simulink model "joint_trajectories"  (R2022a)
settings: Solver=FixedStepAuto  StartTime=0.0  StopTime=inf  RelTol=1e-3
libraries: ros2lib x3
settings Model: Creator=legacy  LastModifiedBy=legacy
settings OptimizationCC: EnhancedBackFolding=on  PassReuseOutputArgsAs=Individual arguments  ZeroExternalMemoryAtStartup=off  ZeroInternalMemoryAtStartup=off  MaxStackSize=64  OptimizeBlockOrder=speed  DifferentSizesBufferReuse=on  OptimizationCustomize=off  EfficientTunableParamExpr=on
settings DebuggingCC: ParameterTunabilityLossMsg=error
settings HardwareCC: ProdBitPerLong=64  ProdHWDeviceType=Intel->x86-64 (Linux 64)  UseEmbeddedCoderFeatures=off
settings SFSimCC: MATLABDynamicMemAlloc=off
settings RTWCC: SystemTargetFile=ert.tlc  HardwareBoard=Robot Operating System 2 (ROS 2)  TLCOptions="-aInlineSetEventsForThisBaseRateFcn=TLC_FALSE -aSuppressMultiTaskScheduler=TLC_FALSE  -aRateBasedStepFcn=0"  TemplateMakefile=ert_default_tmf  Toolchain=Colcon Tools  TargetLang=C++
settings CodeAppCC: ForceParamTrailComments=on  IgnoreCustomStorageClasses=off  OperatorAnnotations=on  SimulinkDataObjDesc=on  SFDataObjDesc=on  InsertBlockDesc=on
settings ERTTargetCC: CodeInterfacePackaging=C++ class  SupportNonInlinedSFcns=on  RootIOFormat=Structure reference

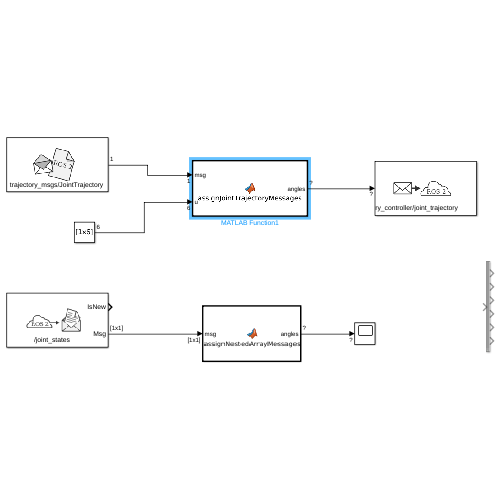
[thumbnail: Simulink's stored preview of the top-level diagram]
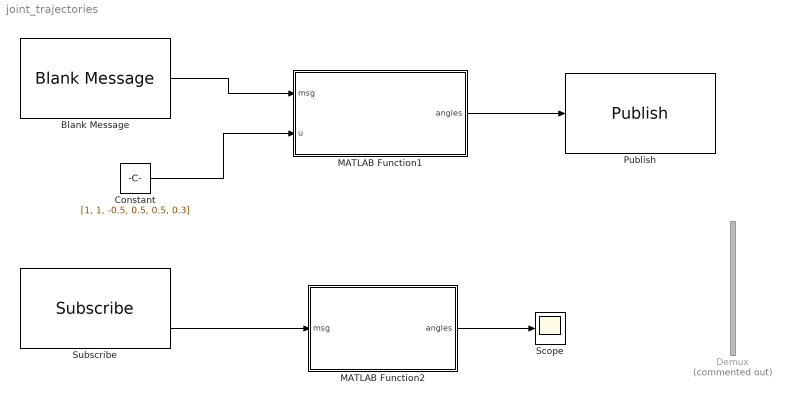
== system joint_trajectories ==
  Blank Message : ros2lib/Blank Message  messageClass=Message  entityType=trajectory_msgs/JointTrajectory  messageType=trajectory_msgs/JointTrajectory  SampleTime=0.01
      settings: SourceProductBaseCode=RR
  Constant : Constant  Value=[1, 1, -0.5, 0.5, 0.5, 0.3]  SampleTime=0.01
  Demux : Demux  Commented=on  Outputs=6
  MATLAB Function1 : MATLAB Function  TreatAsAtomicUnit=on  SystemSampleTime=0.01
  MATLAB Function2 : MATLAB Function  TreatAsAtomicUnit=on  SystemSampleTime=0.01
  Publish : ros2lib/Publish  topicSource=Select from ROS network  topic=/joint_trajectory_controller/joint_trajectory  messageType=trajectory_msgs/JointTrajectory  QOSHistory=Keep last  QOSDepth=1  QOSReliability=Reliable  QOSDurability=Volatile
      settings: SourceProductBaseCode=RR
  Scope : Scope
  Subscribe : ros2lib/Subscribe  topicSource=Select from ROS network  topic=/joint_states  messageType=sensor_msgs/JointState  sampleTime=0.01  QOSHistory=Keep last  QOSDepth=1  QOSReliability=Reliable  QOSDurability=Volatile
      settings: SourceProductBaseCode=RR
  wires:
  Subscribe/2 -> MATLAB Function2/1(msg)
  MATLAB Function2/1(angles) -> Scope/1
  Blank Message/1 -> MATLAB Function1/1(msg)
  Constant/1 -> MATLAB Function1/2(u)
  MATLAB Function1/1(angles) -> Publish/1

== matlab function joint_trajectories/MATLAB Function1 ==
  data: msg input Bus: SL_Bus_trajectory_msgs_JointTrajectory; angles output Bus: SL_Bus_trajectory_msgs_JointTrajectory; u input double
function angles = assignJointTrajectoryMessages(msg, u)
%#codegen

strArrayToAssign = {'joint_base_1', 'joint_12', 'joint_23', 'joint_34', 'joint_45', 'joint_56'};

% Set the number of strings in the string array.
% msg (sensor_msgs/JointState) includes the following fields
%           name : array of std_msgs/String (string array)
%   name_SL_Info : struct with fields CurrentLength, ReceivedLength
numStringsInArray = length(strArrayToAssign);
%msg.name_SL_Info.CurrentLength = uint32(numStringsInArray);

% Set the individual strings in the array
for idx=1:numStringsInArray
    str = strArrayToAssign{idx};
    strLength = length(str);
    msg.joint_names(idx).data(1:strLength) = uint8(str); % 
    %msg.joint_names(idx).data_SL_Info.CurrentLength = uint32(strLength);
end
initial_pos = zeros(1,6);
msg.points.positions(0) = initial_pos;
msg.points.positions(1) = u;

== matlab function joint_trajectories/MATLAB Function2 ==
  data: msg input Bus: SL_Bus_sensor_msgs_JointState; angles output double
function angles = assignNestedArrayMessages(msg)
%#codegen
th1 = msg.position(1);
th2 = msg.position(2);
th3 = msg.position(3);
th4 = msg.position(4);
th5 = msg.position(5);
th6 = msg.position(6);

angles = [th1, th2, th3, th4, th5, th6];
